simulink model "Nadajnik_pluto_qpsk"  (R2024b)
settings: Solver=FixedStepDiscrete  StartTime=0.0  StopTime=inf  RelTol=1e-3
undefined symbols (not defined in the file or in its folder): f, Fs, ip, usb
libraries: plutoradiolib x1, commfilt2 x1, commdigbbndpm3 x1, dspsigops x1
settings Model: Creator=Pinkman  LastModifiedBy=Pinkman
settings SolverCC: AutoInsertRateTranBlk=on
settings DebuggingCC: UnderSpecifiedDimensionMsg=warning

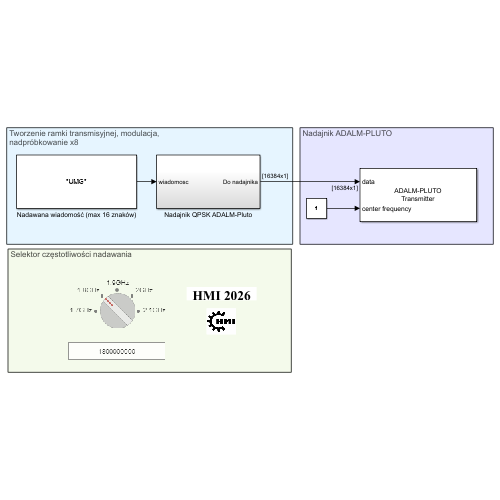
[thumbnail: Simulink's stored preview of the top-level diagram]
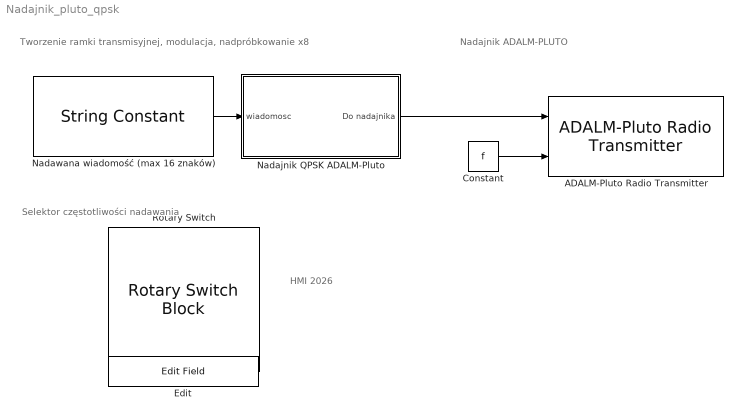
== system Nadajnik_pluto_qpsk ==
  note: Selektor częstotliwości nadawania
  note: Nadajnik ADALM-PLUTO
  note: Tworzenie ramki transmisyjnej, modulacja,
      | nadpróbkowanie x8
  note: HMI 2026
  ADALM-Pluto Radio Transmitter : plutoradiolib/ADALM-Pluto Radio Transmitter  RadioID=usb:1  uri=ip:10.0.0.200  CenterFrequencySource=Input Port  CenterFrequency=f  GainSource=Dialog  Gain=0  ChannelMapping=1  BasebandSampleRate=200e3  UnderflowOutputPort=off  ShowAdvancedProperties=off  UseCustomFilter=off  filtPathRates=[737280000 11520000 3840000 1920000 960000 240000]  filtCoefficients=[-192 82 85 -215 228 -102 -110 290 -318 145 160 -426 471 -215 -238 633 -697 318 349 -923 1009 -457 -498 1309 -1423 640 693 -1812 1959 -876 -945 2458 -2647 1180 1268 -3290 3534 -1572 -1688 4375 -4698 2091 2247 -5836 6284 -2807 -3031 7918 -8588 3870 4225 -11182 12324 -5662 -6330 17255 -19735 9507 11312 -33568 43355 -25227 -42139 305542 305542 -42139 -25227 43355 -33568 11312 9507 -19735 17255 -6330 -5662 12324 -11182 4225 3870 -8588 7918 -3031 -2807 6284 -5836 2247 2091 -4698 4375 -1688 -1572 3534 -3290 1268 1180 -2647 2458 -945 -876 1959 -1812 693 640 -1423 1309 -498 -457 1009 -923 349 318 -697 633 -238 -215 471 -426 160 145 -318 290 -110 -102 228 -215 85 82 -192]  filtCoefficientSize=128  filtDecimInterpFactor=4  filtGain=-12  filtRFBandwidth=18000000  filterConfigStruct=struct()  DataSourceSelect=Input Port  DDSTone1Freq=5e3  DDSTone2Freq=10e3  DDSTone1Scale=0.5  DDSTone2Scale=0.25  DataTimeout=Inf  FrequencyCorrection=0  ENSMPinControlMode=None  BISTLoopbackMode=Disabled  BISTToneInject=Disabled  BISTSignalGen=PRBS  BISTToneFreq=Fs/32  BISTToneLevel=0
  Constant : Constant  Value=f
  Edit : EditField  LabelPosition=Hide  ShowInitialText=on  Alignment=Center
  Nadajnik QPSK ADALM-Pluto : Subsystem
  Nadawana wiadomość (max 16 znaków) : StringConstant  String="\"UMG\""
  Rotary Switch : RotarySwitchBlock  LabelPosition=Hide
      settings: Values={{'1.7GHz', '1.8GHz', '1.9GHz', '2GHz', '2.1GHz'}, [1700000000 1800000000 1900000000 2000000000 2100000000]}
  wires:
  Nadajnik QPSK ADALM-Pluto/1(Do nadajnika) -> ADALM-Pluto Radio Transmitter/1
  Constant/1 -> ADALM-Pluto Radio Transmitter/2
  Nadawana wiadomość (max 16 znaków)/1 -> Nadajnik QPSK ADALM-Pluto/1(wiadomosc)

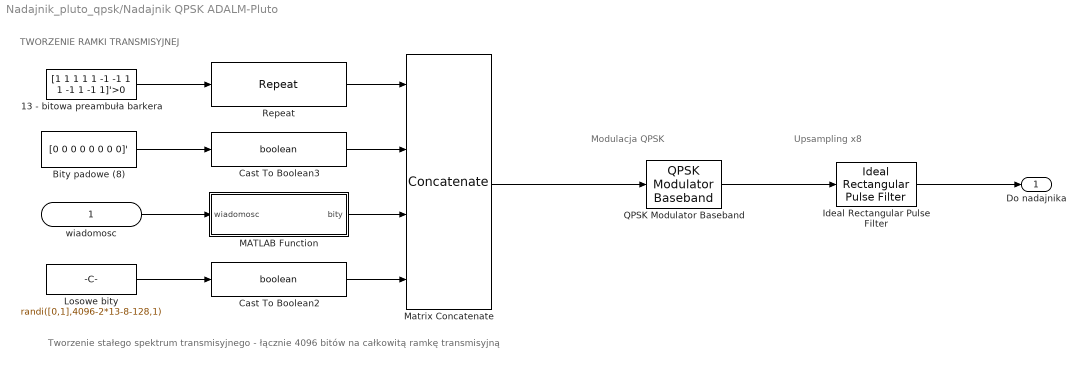
== system Nadajnik_pluto_qpsk/Nadajnik QPSK ADALM-Pluto ==
  note: Upsampling x8
  note: Modulacja QPSK
  note: Tworzenie stałego spektrum transmisyjnego - łącznie 4096 bitów na całkowitą ramkę transmisyjną
  note: TWORZENIE RAMKI TRANSMISYJNEJ
  wiadomosc : Inport
  13 - bitowa preambuła barkera : Constant  Value="[1  1  1  1  1  -1  -1   1   1  -1   1  -1  1]'>0"  VectorParams1D=off
  Bity padowe (8) : Constant  Value=[0 0 0 0 0 0 0 0]'  VectorParams1D=off
  Cast To Boolean2 : DataTypeConversion  OutDataTypeStr=boolean  SaturateOnIntegerOverflow=off  RndMeth=Floor
  Cast To Boolean3 : DataTypeConversion  OutDataTypeStr=boolean  SaturateOnIntegerOverflow=off  RndMeth=Floor
  Ideal Rectangular Pulse Filter : commfilt2/Ideal Rectangular Pulse Filter  pulseLen=8  pulseDelay=0  InputProcessing=Columns as channels (frame based)  RateOptions=Enforce single-rate processing  sampMode=Mute  normCheck=off  normMode=Sum of samples  filterGain=1  saveAsFlag=0  roundingMode=Floor  overflowMode=off  firstCoeffDataTypeStr=Inherit: Same word length as input  firstCoeffMin=[]  firstCoeffMax=[]  firstCoeffLastDataTypeStr=Inherit: Same word length as input  outputDataTypeStr=Inherit: Same as accumulator  outputMin=[]  outputMax=[]  outputLastDataTypeStr=Inherit: Same as accumulator
  Losowe bity : Constant  Value=randi([0,1],4096-2*13-8-128,1)
  MATLAB Function : MATLAB Function  TreatAsAtomicUnit=on
  Matrix Concatenate : Concatenate  NumInputs=4  Mode=Multidimensional array
  QPSK Modulator Baseband : commdigbbndpm3/QPSK Modulator Baseband  InType=Bit  Enc=Gray  Ph=pi/4  outDtype=double  outWordLen=16  outUDDataType=sfix(16)  outFracLenMode=Best precision  outFracLen=15  outDataTypeStr=double  outLastDataTypeStr=double
      settings: LibrarySourceBlock=|
      | commhdldigbbndpm/QPSK
      | Modulator
      | Baseband
  Repeat : dspsigops/Repeat  FactorSource=Dialog parameter  N=2  Nmax=16  InputProcessing=Columns as channels (frame based)  RateOptions=Enforce single-rate processing  ic=0  mode=Unused parameter value
      settings: LibrarySourceBlock=commsequence2/Repeat
  Do nadajnika : Outport
  wires:
  QPSK Modulator Baseband/1 -> Ideal Rectangular Pulse Filter/1
  Matrix Concatenate/1 -> QPSK Modulator Baseband/1
  Ideal Rectangular Pulse Filter/1 -> Do nadajnika/1
  13 - bitowa preambuła barkera/1 -> Repeat/1
  Repeat/1 -> Matrix Concatenate/1
  Bity padowe (8)/1 -> Cast To Boolean3/1
  Losowe bity/1 -> Cast To Boolean2/1
  MATLAB Function/1(bity) -> Matrix Concatenate/3
  Cast To Boolean2/1 -> Matrix Concatenate/4
  Cast To Boolean3/1 -> Matrix Concatenate/2
  wiadomosc/1 -> MATLAB Function/1(wiadomosc)

== matlab function Nadajnik_pluto_qpsk/Nadajnik QPSK ADALM-Pluto/MATLAB Function ==
  data: bity output; wiadomosc input
function bity =  transmisja(wiadomosc)

MAX_DLU = 128; 

bity = false(MAX_DLU, 1); 
     
temp_bity = boolean(int2bit(double(char(wiadomosc))',8));
      
dl = length(temp_bity);
if dl > MAX_DLU
    error("Wiadomość za długa, max to 128 znaków.");
end

bity(1:dl) = temp_bity;
